simulink model "VCU_CS75_10_9_SteeringTorque"  (R2014a)
settings: Solver=FixedStepDiscrete  StartTime=0.0  StopTime=25  FixedStep=0.0005  RelTol=1e-3
undefined symbols (not defined in the file or in its folder): AutoDrivingReady, ecucoder_acal, I_SW01_L, LaterlAngleCommand, LDW, RemoteAcclPosition
libraries: simulink x880, ec5744lib x37
(part 15 of 30)

== system VCU_CS75_10_9_SteeringTorque/长安CS75底盘程序，20ms一次/Output/CAN1_Tx/to28D/LAS_28D/LAS_LDWReminder ==
  LAS_LDWReminder : Inport
  Constant{1..2,4..8} (7 alike) : Constant  Value=0  OutDataTypeStr=uint8
  LAS_LDWReminderRon : Rounding  Operator=round
  LAS_LDWReminder_1sat : Saturate  UpperLimit=96  LowerLimit=0
  LAS_LDWReminder_Convert : DataTypeConversion  OutDataTypeStr=uint8
  LAS_LDWReminder_Convert1 : DataTypeConversion  OutDataTypeStr=uint32
  LAS_LDWReminder_D : Product  Inputs=*/
  LAS_LDWReminder_F : Constant  OutDataTypeStr=single
  LAS_LDWReminder_L : simulink/Logic and Bit Operations/Bitwise Operator  logicop=AND  UseBitMask=on  BitMask=96  BitMaskRealWorld=Stored Integer
  LAS_LDWReminder_O : Constant  Value=0  OutDataTypeStr=single
  LAS_LDWReminder_S : ArithShift  BitShiftNumber=-5
  LAS_LDWReminder_sat : Saturate  UpperLimit=0  LowerLimit=0
  LAS_LDWReminder_st : Sum  Inputs=+-
  output1 : Outport
  output2 : Outport  Port=2
  output3 : Outport  Port=3
  output4 : Outport  Port=4
  output5 : Outport  Port=5
  output6 : Outport  Port=6
  output7 : Outport  Port=7
  output8 : Outport  Port=8
  wires:
  LAS_LDWReminder/1 -> LAS_LDWReminder_sat/1
  LAS_LDWReminder_sat/1 -> LAS_LDWReminder_st/1
  LAS_LDWReminder_O/1 -> LAS_LDWReminder_st/2
  LAS_LDWReminder_st/1 -> LAS_LDWReminder_D/1
  LAS_LDWReminder_F/1 -> LAS_LDWReminder_D/2
  LAS_LDWReminder_D/1 -> LAS_LDWReminderRon/1
  LAS_LDWReminderRon/1 -> LAS_LDWReminder_S/1
  LAS_LDWReminder_S/1 -> LAS_LDWReminder_1sat/1
  LAS_LDWReminder_1sat/1 -> LAS_LDWReminder_Convert1/1
  LAS_LDWReminder_Convert1/1 -> LAS_LDWReminder_L/1
  LAS_LDWReminder_L/1 -> LAS_LDWReminder_Convert/1
  LAS_LDWReminder_Convert/1 -> output3/1
  Constant1/1 -> output1/1
  Constant2/1 -> output2/1
  Constant4/1 -> output4/1
  Constant5/1 -> output5/1
  Constant6/1 -> output6/1
  Constant7/1 -> output7/1
  Constant8/1 -> output8/1

== system VCU_CS75_10_9_SteeringTorque/长安CS75底盘程序，20ms一次/Output/CAN1_Tx/to28D/LAS_28D/LAS_LDWStatus ==
  LAS_LDWStatus : Inport
  Constant{2..8} (7 alike) : Constant  Value=0  OutDataTypeStr=uint8
  LAS_LDWStatusRon : Rounding  Operator=round
  LAS_LDWStatus_1sat : Saturate  UpperLimit=96  LowerLimit=0
  LAS_LDWStatus_Convert : DataTypeConversion  OutDataTypeStr=uint8
  LAS_LDWStatus_Convert1 : DataTypeConversion  OutDataTypeStr=uint32
  LAS_LDWStatus_D : Product  Inputs=*/
  LAS_LDWStatus_F : Constant  OutDataTypeStr=single
  LAS_LDWStatus_L : simulink/Logic and Bit Operations/Bitwise Operator  logicop=AND  UseBitMask=on  BitMask=96  BitMaskRealWorld=Stored Integer
  LAS_LDWStatus_O : Constant  Value=0  OutDataTypeStr=single
  LAS_LDWStatus_S : ArithShift  BitShiftNumber=-5
  LAS_LDWStatus_sat : Saturate  UpperLimit=3  LowerLimit=0
  LAS_LDWStatus_st : Sum  Inputs=+-
  output1 : Outport
  output2 : Outport  Port=2
  output3 : Outport  Port=3
  output4 : Outport  Port=4
  output5 : Outport  Port=5
  output6 : Outport  Port=6
  output7 : Outport  Port=7
  output8 : Outport  Port=8
  wires:
  LAS_LDWStatus/1 -> LAS_LDWStatus_sat/1
  LAS_LDWStatus_sat/1 -> LAS_LDWStatus_st/1
  LAS_LDWStatus_O/1 -> LAS_LDWStatus_st/2
  LAS_LDWStatus_st/1 -> LAS_LDWStatus_D/1
  LAS_LDWStatus_F/1 -> LAS_LDWStatus_D/2
  LAS_LDWStatus_D/1 -> LAS_LDWStatusRon/1
  LAS_LDWStatusRon/1 -> LAS_LDWStatus_S/1
  LAS_LDWStatus_S/1 -> LAS_LDWStatus_1sat/1
  LAS_LDWStatus_1sat/1 -> LAS_LDWStatus_Convert1/1
  LAS_LDWStatus_Convert1/1 -> LAS_LDWStatus_L/1
  LAS_LDWStatus_L/1 -> LAS_LDWStatus_Convert/1
  LAS_LDWStatus_Convert/1 -> output1/1
  Constant2/1 -> output2/1
  Constant3/1 -> output3/1
  Constant4/1 -> output4/1
  Constant5/1 -> output5/1
  Constant6/1 -> output6/1
  Constant7/1 -> output7/1
  Constant8/1 -> output8/1

== system VCU_CS75_10_9_SteeringTorque/长安CS75底盘程序，20ms一次/Output/CAN1_Tx/to28D/LAS_28D/LAS_LDWVibrationWarning ==
  LAS_LDWVibrationWarning : Inport
  Constant{1,3..8} (7 alike) : Constant  Value=0  OutDataTypeStr=uint8
  LAS_LDWVibrationWarningRon : Rounding  Operator=round
  LAS_LDWVibrationWarning_1sat : Saturate  UpperLimit=96  LowerLimit=0
  LAS_LDWVibrationWarning_Convert : DataTypeConversion  OutDataTypeStr=uint8
  LAS_LDWVibrationWarning_Convert1 : DataTypeConversion  OutDataTypeStr=uint32
  LAS_LDWVibrationWarning_D : Product  Inputs=*/
  LAS_LDWVibrationWarning_F : Constant  OutDataTypeStr=single
  LAS_LDWVibrationWarning_L : simulink/Logic and Bit Operations/Bitwise Operator  logicop=AND  UseBitMask=on  BitMask=96  BitMaskRealWorld=Stored Integer
  LAS_LDWVibrationWarning_O : Constant  Value=0  OutDataTypeStr=single
  LAS_LDWVibrationWarning_S : ArithShift  BitShiftNumber=-5
  LAS_LDWVibrationWarning_sat : Saturate  UpperLimit=3  LowerLimit=0
  LAS_LDWVibrationWarning_st : Sum  Inputs=+-
  output1 : Outport
  output2 : Outport  Port=2
  output3 : Outport  Port=3
  output4 : Outport  Port=4
  output5 : Outport  Port=5
  output6 : Outport  Port=6
  output7 : Outport  Port=7
  output8 : Outport  Port=8
  wires:
  LAS_LDWVibrationWarning/1 -> LAS_LDWVibrationWarning_sat/1
  LAS_LDWVibrationWarning_sat/1 -> LAS_LDWVibrationWarning_st/1
  LAS_LDWVibrationWarning_O/1 -> LAS_LDWVibrationWarning_st/2
  LAS_LDWVibrationWarning_st/1 -> LAS_LDWVibrationWarning_D/1
  LAS_LDWVibrationWarning_F/1 -> LAS_LDWVibrationWarning_D/2
  LAS_LDWVibrationWarning_D/1 -> LAS_LDWVibrationWarningRon/1
  LAS_LDWVibrationWarningRon/1 -> LAS_LDWVibrationWarning_S/1
  LAS_LDWVibrationWarning_S/1 -> LAS_LDWVibrationWarning_1sat/1
  LAS_LDWVibrationWarning_1sat/1 -> LAS_LDWVibrationWarning_Convert1/1
  LAS_LDWVibrationWarning_Convert1/1 -> LAS_LDWVibrationWarning_L/1
  LAS_LDWVibrationWarning_L/1 -> LAS_LDWVibrationWarning_Convert/1
  LAS_LDWVibrationWarning_Convert/1 -> output2/1
  Constant1/1 -> output1/1
  Constant3/1 -> output3/1
  Constant4/1 -> output4/1
  Constant5/1 -> output5/1
  Constant6/1 -> output6/1
  Constant7/1 -> output7/1
  Constant8/1 -> output8/1

== system VCU_CS75_10_9_SteeringTorque/长安CS75底盘程序，20ms一次/Output/CAN1_Tx/to28D/LAS_28D/LAS_LKSStatus ==
  LAS_LKSStatus : Inport
  Constant{1..4,6..8} (7 alike) : Constant  Value=0  OutDataTypeStr=uint8
  LAS_LKSStatusRon : Rounding  Operator=round
  LAS_LKSStatus_1sat : Saturate  UpperLimit=224  LowerLimit=0
  LAS_LKSStatus_Convert : DataTypeConversion  OutDataTypeStr=uint8
  LAS_LKSStatus_Convert1 : DataTypeConversion  OutDataTypeStr=uint32
  LAS_LKSStatus_D : Product  Inputs=*/
  LAS_LKSStatus_F : Constant  OutDataTypeStr=single
  LAS_LKSStatus_L : simulink/Logic and Bit Operations/Bitwise Operator  logicop=AND  UseBitMask=on  BitMask=224  BitMaskRealWorld=Stored Integer
  LAS_LKSStatus_O : Constant  Value=0  OutDataTypeStr=single
  LAS_LKSStatus_S : ArithShift  BitShiftNumber=-5
  LAS_LKSStatus_sat : Saturate  UpperLimit=7  LowerLimit=0
  LAS_LKSStatus_st : Sum  Inputs=+-
  output1 : Outport
  output2 : Outport  Port=2
  output3 : Outport  Port=3
  output4 : Outport  Port=4
  output5 : Outport  Port=5
  output6 : Outport  Port=6
  output7 : Outport  Port=7
  output8 : Outport  Port=8
  wires:
  LAS_LKSStatus/1 -> LAS_LKSStatus_sat/1
  LAS_LKSStatus_sat/1 -> LAS_LKSStatus_st/1
  LAS_LKSStatus_O/1 -> LAS_LKSStatus_st/2
  LAS_LKSStatus_st/1 -> LAS_LKSStatus_D/1
  LAS_LKSStatus_F/1 -> LAS_LKSStatus_D/2
  LAS_LKSStatus_D/1 -> LAS_LKSStatusRon/1
  LAS_LKSStatusRon/1 -> LAS_LKSStatus_S/1
  LAS_LKSStatus_S/1 -> LAS_LKSStatus_1sat/1
  LAS_LKSStatus_1sat/1 -> LAS_LKSStatus_Convert1/1
  LAS_LKSStatus_Convert1/1 -> LAS_LKSStatus_L/1
  LAS_LKSStatus_L/1 -> LAS_LKSStatus_Convert/1
  LAS_LKSStatus_Convert/1 -> output5/1
  Constant1/1 -> output1/1
  Constant2/1 -> output2/1
  Constant3/1 -> output3/1
  Constant4/1 -> output4/1
  Constant6/1 -> output6/1
  Constant7/1 -> output7/1
  Constant8/1 -> output8/1

== system VCU_CS75_10_9_SteeringTorque/长安CS75底盘程序，20ms一次/Output/CAN1_Tx/to28D/LAS_28D/LAS_SLASpdLimit ==
  LAS_SLASpdLimit : Inport
  Constant{1..2,5..8} (6 alike) : Constant  Value=0  OutDataTypeStr=uint8
  LAS_SLASpdLimitBitCov : DataTypeConversion  OutDataTypeStr=uint8
  LAS_SLASpdLimitCOV : DataTypeConversion  OutDataTypeStr=uint8
  LAS_SLASpdLimitRon : Rounding  Operator=round
  LAS_SLASpdLimit_1sat : Saturate  UpperLimit=4080  LowerLimit=0
  LAS_SLASpdLimit_And : simulink/Logic and Bit Operations/Bitwise Operator  logicop=AND  UseBitMask=off  NumInputPorts=2  BitMask=bin2dec('11011001')  BitMaskRealWorld=Stored Integer
  LAS_SLASpdLimit_And_C : Constant  Value=255  OutDataTypeStr=uint32
  LAS_SLASpdLimit_Convert : DataTypeConversion  OutDataTypeStr=uint32
  LAS_SLASpdLimit_D : Product  Inputs=*/
  LAS_SLASpdLimit_D1 : Product  Inputs=*/
  LAS_SLASpdLimit_F : Constant  OutDataTypeStr=single
  LAS_SLASpdLimit_L : simulink/Logic and Bit Operations/Bitwise Operator  logicop=AND  UseBitMask=on  BitMask=4080  BitMaskRealWorld=Stored Integer
  LAS_SLASpdLimit_O : Constant  Value=0  OutDataTypeStr=single
  LAS_SLASpdLimit_S : ArithShift  BitShiftNumber=-4
  LAS_SLASpdLimit_sat : Saturate  UpperLimit=0  LowerLimit=0
  LAS_SLASpdLimit_st : Sum  Inputs=+-
  LAS_SLASpdLimitoutput3_C : Constant  Value=256
  output1 : Outport
  output2 : Outport  Port=2
  output3 : Outport  Port=3
  output4 : Outport  Port=4
  output5 : Outport  Port=5
  output6 : Outport  Port=6
  output7 : Outport  Port=7
  output8 : Outport  Port=8
  wires:
  LAS_SLASpdLimit/1 -> LAS_SLASpdLimit_sat/1
  LAS_SLASpdLimit_sat/1 -> LAS_SLASpdLimit_st/1
  LAS_SLASpdLimit_O/1 -> LAS_SLASpdLimit_st/2
  LAS_SLASpdLimit_st/1 -> LAS_SLASpdLimit_D/1
  LAS_SLASpdLimit_F/1 -> LAS_SLASpdLimit_D/2
  LAS_SLASpdLimit_D/1 -> LAS_SLASpdLimitRon/1
  LAS_SLASpdLimitRon/1 -> LAS_SLASpdLimit_S/1
  LAS_SLASpdLimit_S/1 -> LAS_SLASpdLimit_1sat/1
  LAS_SLASpdLimit_1sat/1 -> LAS_SLASpdLimit_Convert/1
  LAS_SLASpdLimit_Convert/1 -> LAS_SLASpdLimit_L/1
  LAS_SLASpdLimit_L/1 -> LAS_SLASpdLimit_D1/1, LAS_SLASpdLimit_And/1
  LAS_SLASpdLimitoutput3_C/1 -> LAS_SLASpdLimit_D1/2
  LAS_SLASpdLimit_D1/1 -> LAS_SLASpdLimitCOV/1
  LAS_SLASpdLimitCOV/1 -> output3/1
  LAS_SLASpdLimit_And_C/1 -> LAS_SLASpdLimit_And/2
  LAS_SLASpdLimit_And/1 -> LAS_SLASpdLimitBitCov/1
  LAS_SLASpdLimitBitCov/1 -> output4/1
  Constant1/1 -> output1/1
  Constant2/1 -> output2/1
  Constant5/1 -> output5/1
  Constant6/1 -> output6/1
  Constant7/1 -> output7/1
  Constant8/1 -> output8/1

== system VCU_CS75_10_9_SteeringTorque/长安CS75底盘程序，20ms一次/Output/CAN1_Tx/to28D/LAS_28D/LAS_SLASpdLimitUnit ==
  LAS_SLASpdLimitUnit : Inport
  Constant{2..8} (7 alike) : Constant  Value=0  OutDataTypeStr=uint8
  LAS_SLASpdLimitUnitRon : Rounding  Operator=round
  LAS_SLASpdLimitUnit_1sat : Saturate  UpperLimit=12  LowerLimit=0
  LAS_SLASpdLimitUnit_Convert : DataTypeConversion  OutDataTypeStr=uint8
  LAS_SLASpdLimitUnit_Convert1 : DataTypeConversion  OutDataTypeStr=uint32
  LAS_SLASpdLimitUnit_D : Product  Inputs=*/
  LAS_SLASpdLimitUnit_F : Constant  OutDataTypeStr=single
  LAS_SLASpdLimitUnit_L : simulink/Logic and Bit Operations/Bitwise Operator  logicop=AND  UseBitMask=on  BitMask=12  BitMaskRealWorld=Stored Integer
  LAS_SLASpdLimitUnit_O : Constant  Value=0  OutDataTypeStr=single
  LAS_SLASpdLimitUnit_S : ArithShift  BitShiftNumber=-2
  LAS_SLASpdLimitUnit_sat : Saturate  UpperLimit=0  LowerLimit=0
  LAS_SLASpdLimitUnit_st : Sum  Inputs=+-
  output1 : Outport
  output2 : Outport  Port=2
  output3 : Outport  Port=3
  output4 : Outport  Port=4
  output5 : Outport  Port=5
  output6 : Outport  Port=6
  output7 : Outport  Port=7
  output8 : Outport  Port=8
  wires:
  LAS_SLASpdLimitUnit/1 -> LAS_SLASpdLimitUnit_sat/1
  LAS_SLASpdLimitUnit_sat/1 -> LAS_SLASpdLimitUnit_st/1
  LAS_SLASpdLimitUnit_O/1 -> LAS_SLASpdLimitUnit_st/2
  LAS_SLASpdLimitUnit_st/1 -> LAS_SLASpdLimitUnit_D/1
  LAS_SLASpdLimitUnit_F/1 -> LAS_SLASpdLimitUnit_D/2
  LAS_SLASpdLimitUnit_D/1 -> LAS_SLASpdLimitUnitRon/1
  LAS_SLASpdLimitUnitRon/1 -> LAS_SLASpdLimitUnit_S/1
  LAS_SLASpdLimitUnit_S/1 -> LAS_SLASpdLimitUnit_1sat/1
  LAS_SLASpdLimitUnit_1sat/1 -> LAS_SLASpdLimitUnit_Convert1/1
  LAS_SLASpdLimitUnit_Convert1/1 -> LAS_SLASpdLimitUnit_L/1
  LAS_SLASpdLimitUnit_L/1 -> LAS_SLASpdLimitUnit_Convert/1
  LAS_SLASpdLimitUnit_Convert/1 -> output1/1
  Constant2/1 -> output2/1
  Constant3/1 -> output3/1
  Constant4/1 -> output4/1
  Constant5/1 -> output5/1
  Constant6/1 -> output6/1
  Constant7/1 -> output7/1
  Constant8/1 -> output8/1

== system VCU_CS75_10_9_SteeringTorque/长安CS75底盘程序，20ms一次/Output/CAN1_Tx/to28D/LAS_28D/LAS_SLAState ==
  LAS_SLAState : Inport
  Constant{1..4,6..8} (7 alike) : Constant  Value=0  OutDataTypeStr=uint8
  LAS_SLAStateRon : Rounding  Operator=round
  LAS_SLAState_1sat : Saturate  UpperLimit=28  LowerLimit=0
  LAS_SLAState_Convert : DataTypeConversion  OutDataTypeStr=uint8
  LAS_SLAState_Convert1 : DataTypeConversion  OutDataTypeStr=uint32
  LAS_SLAState_D : Product  Inputs=*/
  LAS_SLAState_F : Constant  OutDataTypeStr=single
  LAS_SLAState_L : simulink/Logic and Bit Operations/Bitwise Operator  logicop=AND  UseBitMask=on  BitMask=28  BitMaskRealWorld=Stored Integer
  LAS_SLAState_O : Constant  Value=0  OutDataTypeStr=single
  LAS_SLAState_S : ArithShift  BitShiftNumber=-2
  LAS_SLAState_sat : Saturate  UpperLimit=0  LowerLimit=0
  LAS_SLAState_st : Sum  Inputs=+-
  output1 : Outport
  output2 : Outport  Port=2
  output3 : Outport  Port=3
  output4 : Outport  Port=4
  output5 : Outport  Port=5
  output6 : Outport  Port=6
  output7 : Outport  Port=7
  output8 : Outport  Port=8
  wires:
  LAS_SLAState/1 -> LAS_SLAState_sat/1
  LAS_SLAState_sat/1 -> LAS_SLAState_st/1
  LAS_SLAState_O/1 -> LAS_SLAState_st/2
  LAS_SLAState_st/1 -> LAS_SLAState_D/1
  LAS_SLAState_F/1 -> LAS_SLAState_D/2
  LAS_SLAState_D/1 -> LAS_SLAStateRon/1
  LAS_SLAStateRon/1 -> LAS_SLAState_S/1
  LAS_SLAState_S/1 -> LAS_SLAState_1sat/1
  LAS_SLAState_1sat/1 -> LAS_SLAState_Convert1/1
  LAS_SLAState_Convert1/1 -> LAS_SLAState_L/1
  LAS_SLAState_L/1 -> LAS_SLAState_Convert/1
  LAS_SLAState_Convert/1 -> output5/1
  Constant1/1 -> output1/1
  Constant2/1 -> output2/1
  Constant3/1 -> output3/1
  Constant4/1 -> output4/1
  Constant6/1 -> output6/1
  Constant7/1 -> output7/1
  Constant8/1 -> output8/1

== system VCU_CS75_10_9_SteeringTorque/长安CS75底盘程序，20ms一次/Output/CAN1_Tx/to28D/LAS_28D/LAS_SteeringTorqueReq ==
  LAS_SteeringTorqueReq : Inport
  Constant{1..4,8} (5 alike) : Constant  Value=0  OutDataTypeStr=uint8
  LAS_SteeringTorqueReqBitCov : DataTypeConversion  OutDataTypeStr=uint32
  LAS_SteeringTorqueReqBitCov1 : DataTypeConversion  OutDataTypeStr=uint8
  LAS_SteeringTorqueReqCOV : DataTypeConversion  OutDataTypeStr=uint8
  LAS_SteeringTorqueReqCOV1 : DataTypeConversion  OutDataTypeStr=uint8
  LAS_SteeringTorqueReqRon : Rounding  Operator=round
  LAS_SteeringTorqueReq_1sat : Saturate  UpperLimit=262016  LowerLimit=0
  LAS_SteeringTorqueReq_And : simulink/Logic and Bit Operations/Bitwise Operator  logicop=AND  UseBitMask=off  NumInputPorts=2  BitMask=bin2dec('11011001')  BitMaskRealWorld=Stored Integer
  LAS_SteeringTorqueReq_And1 : simulink/Logic and Bit Operations/Bitwise Operator  logicop=AND  UseBitMask=off  NumInputPorts=2  BitMask=bin2dec('11011001')  BitMaskRealWorld=Stored Integer
  LAS_SteeringTorqueReq_And1_C : Constant  Value=255  OutDataTypeStr=uint32
  LAS_SteeringTorqueReq_And_C : Constant  Value=65535
  LAS_SteeringTorqueReq_Convert : DataTypeConversion  OutDataTypeStr=uint32
  LAS_SteeringTorqueReq_D : Product  Inputs=*/
  LAS_SteeringTorqueReq_D1 : Product  Inputs=*/
  LAS_SteeringTorqueReq_D2 : Product  Inputs=*/
  LAS_SteeringTorqueReq_F : Constant  Value=0.01  OutDataTypeStr=single
  LAS_SteeringTorqueReq_L : simulink/Logic and Bit Operations/Bitwise Operator  logicop=AND  UseBitMask=on  BitMask=262016  BitMaskRealWorld=Stored Integer
  LAS_SteeringTorqueReq_O : Constant  Value=-8  OutDataTypeStr=single
  LAS_SteeringTorqueReq_S : ArithShift  BitShiftNumber=-7
  LAS_SteeringTorqueReq_sat : Saturate  UpperLimit=12.47  LowerLimit=-8
  LAS_SteeringTorqueReq_st : Sum  Inputs=+-
  LAS_SteeringTorqueReqoutput5_C : Constant  Value=65536
  LAS_SteeringTorqueReqoutput6_C : Constant  Value=256
  output1 : Outport
  output2 : Outport  Port=2
  output3 : Outport  Port=3
  output4 : Outport  Port=4
  output5 : Outport  Port=5
  output6 : Outport  Port=6
  output7 : Outport  Port=7
  output8 : Outport  Port=8
  wires:
  LAS_SteeringTorqueReq/1 -> LAS_SteeringTorqueReq_sat/1
  LAS_SteeringTorqueReq_sat/1 -> LAS_SteeringTorqueReq_st/1
  LAS_SteeringTorqueReq_O/1 -> LAS_SteeringTorqueReq_st/2
  LAS_SteeringTorqueReq_st/1 -> LAS_SteeringTorqueReq_D/1
  LAS_SteeringTorqueReq_F/1 -> LAS_SteeringTorqueReq_D/2
  LAS_SteeringTorqueReq_D/1 -> LAS_SteeringTorqueReqRon/1
  LAS_SteeringTorqueReqRon/1 -> LAS_SteeringTorqueReq_S/1
  LAS_SteeringTorqueReq_S/1 -> LAS_SteeringTorqueReq_1sat/1
  LAS_SteeringTorqueReq_1sat/1 -> LAS_SteeringTorqueReq_Convert/1
  LAS_SteeringTorqueReq_Convert/1 -> LAS_SteeringTorqueReq_L/1
  LAS_SteeringTorqueReq_L/1 -> LAS_SteeringTorqueReq_D1/1, LAS_SteeringTorqueReq_And/1, LAS_SteeringTorqueReq_And1/1
  LAS_SteeringTorqueReqoutput5_C/1 -> LAS_SteeringTorqueReq_D1/2
  LAS_SteeringTorqueReq_D1/1 -> LAS_SteeringTorqueReqCOV/1
  LAS_SteeringTorqueReqCOV/1 -> output5/1
  LAS_SteeringTorqueReq_And_C/1 -> LAS_SteeringTorqueReqBitCov/1
  LAS_SteeringTorqueReqBitCov/1 -> LAS_SteeringTorqueReq_And/2
  LAS_SteeringTorqueReq_And/1 -> LAS_SteeringTorqueReq_D2/1
  LAS_SteeringTorqueReqoutput6_C/1 -> LAS_SteeringTorqueReq_D2/2
  LAS_SteeringTorqueReq_D2/1 -> LAS_SteeringTorqueReqCOV1/1
  LAS_SteeringTorqueReqCOV1/1 -> output6/1
  LAS_SteeringTorqueReq_And1_C/1 -> LAS_SteeringTorqueReq_And1/2
  LAS_SteeringTorqueReq_And1/1 -> LAS_SteeringTorqueReqBitCov1/1
  LAS_SteeringTorqueReqBitCov1/1 -> output7/1
  Constant1/1 -> output1/1
  Constant2/1 -> output2/1
  Constant3/1 -> output3/1
  Constant4/1 -> output4/1
  Constant8/1 -> output8/1

== system VCU_CS75_10_9_SteeringTorque/长安CS75底盘程序，20ms一次/Output/CAN1_Tx/to28D/LAS_28D/LAS_TakeoverReq ==
  LAS_TakeoverReq : Inport
  Constant{1,3..8} (7 alike) : Constant  Value=0  OutDataTypeStr=uint8
  LAS_TakeoverReqRon : Rounding  Operator=round
  LAS_TakeoverReq_1sat : Saturate  UpperLimit=4  LowerLimit=0
  LAS_TakeoverReq_Convert : DataTypeConversion  OutDataTypeStr=uint8
  LAS_TakeoverReq_Convert1 : DataTypeConversion  OutDataTypeStr=uint32
  LAS_TakeoverReq_D : Product  Inputs=*/
  LAS_TakeoverReq_F : Constant  OutDataTypeStr=single
  LAS_TakeoverReq_L : simulink/Logic and Bit Operations/Bitwise Operator  logicop=AND  UseBitMask=on  BitMask=4  BitMaskRealWorld=Stored Integer
  LAS_TakeoverReq_O : Constant  Value=0  OutDataTypeStr=single
  LAS_TakeoverReq_S : ArithShift  BitShiftNumber=-2
  LAS_TakeoverReq_sat : Saturate  UpperLimit=1  LowerLimit=0
  LAS_TakeoverReq_st : Sum  Inputs=+-
  output1 : Outport
  output2 : Outport  Port=2
  output3 : Outport  Port=3
  output4 : Outport  Port=4
  output5 : Outport  Port=5
  output6 : Outport  Port=6
  output7 : Outport  Port=7
  output8 : Outport  Port=8
  wires:
  LAS_TakeoverReq/1 -> LAS_TakeoverReq_sat/1
  LAS_TakeoverReq_sat/1 -> LAS_TakeoverReq_st/1
  LAS_TakeoverReq_O/1 -> LAS_TakeoverReq_st/2
  LAS_TakeoverReq_st/1 -> LAS_TakeoverReq_D/1
  LAS_TakeoverReq_F/1 -> LAS_TakeoverReq_D/2
  LAS_TakeoverReq_D/1 -> LAS_TakeoverReqRon/1
  LAS_TakeoverReqRon/1 -> LAS_TakeoverReq_S/1
  LAS_TakeoverReq_S/1 -> LAS_TakeoverReq_1sat/1
  LAS_TakeoverReq_1sat/1 -> LAS_TakeoverReq_Convert1/1
  LAS_TakeoverReq_Convert1/1 -> LAS_TakeoverReq_L/1
  LAS_TakeoverReq_L/1 -> LAS_TakeoverReq_Convert/1
  LAS_TakeoverReq_Convert/1 -> output2/1
  Constant1/1 -> output1/1
  Constant3/1 -> output3/1
  Constant4/1 -> output4/1
  Constant5/1 -> output5/1
  Constant6/1 -> output6/1
  Constant7/1 -> output7/1
  Constant8/1 -> output8/1

== system VCU_CS75_10_9_SteeringTorque/长安CS75底盘程序，20ms一次/Output/CAN1_Tx/to28D/LAS_28D/RollingConter ==
  RollingConter : Inport
  Constant{1..6,8} (7 alike) : Constant  Value=0  OutDataTypeStr=uint8
  RollingConterRon : Rounding  Operator=round
  RollingConter_1sat : Saturate  UpperLimit=15  LowerLimit=0
  RollingConter_Convert : DataTypeConversion  OutDataTypeStr=uint8
  RollingConter_Convert1 : DataTypeConversion  OutDataTypeStr=uint32
  RollingConter_D : Product  Inputs=*/
  RollingConter_F : Constant  OutDataTypeStr=single
  RollingConter_L : simulink/Logic and Bit Operations/Bitwise Operator  logicop=AND  UseBitMask=on  BitMask=15  BitMaskRealWorld=Stored Integer
  RollingConter_O : Constant  Value=0  OutDataTypeStr=single
  RollingConter_S : ArithShift
  RollingConter_sat : Saturate  UpperLimit=15  LowerLimit=0
  RollingConter_st : Sum  Inputs=+-
  output1 : Outport
  output2 : Outport  Port=2
  output3 : Outport  Port=3
  output4 : Outport  Port=4
  output5 : Outport  Port=5
  output6 : Outport  Port=6
  output7 : Outport  Port=7
  output8 : Outport  Port=8
  wires:
  RollingConter/1 -> RollingConter_sat/1
  RollingConter_sat/1 -> RollingConter_st/1
  RollingConter_O/1 -> RollingConter_st/2
  RollingConter_st/1 -> RollingConter_D/1
  RollingConter_F/1 -> RollingConter_D/2
  RollingConter_D/1 -> RollingConterRon/1
  RollingConterRon/1 -> RollingConter_S/1
  RollingConter_S/1 -> RollingConter_1sat/1
  RollingConter_1sat/1 -> RollingConter_Convert1/1
  RollingConter_Convert1/1 -> RollingConter_L/1
  RollingConter_L/1 -> RollingConter_Convert/1
  RollingConter_Convert/1 -> output7/1
  Constant1/1 -> output1/1
  Constant2/1 -> output2/1
  Constant3/1 -> output3/1
  Constant4/1 -> output4/1
  Constant5/1 -> output5/1
  Constant6/1 -> output6/1
  Constant8/1 -> output8/1

== system VCU_CS75_10_9_SteeringTorque/长安CS75底盘程序，20ms一次/Output/CAN1_Tx/to2E4/ACC_2E4/ACC_ACCTargetAcceleration ==
  ACC_ACCTargetAcceleration : Inport
  ACC_ACCTargetAccelerationRon : Rounding  Operator=round
  ACC_ACCTargetAcceleration_1sat : Saturate  UpperLimit=255  LowerLimit=0
  ACC_ACCTargetAcceleration_Convert : DataTypeConversion  OutDataTypeStr=uint8
  ACC_ACCTargetAcceleration_Convert1 : DataTypeConversion  OutDataTypeStr=uint32
  ACC_ACCTargetAcceleration_D : Product  Inputs=*/
  ACC_ACCTargetAcceleration_F : Constant  Value=0.05  OutDataTypeStr=single
  ACC_ACCTargetAcceleration_L : simulink/Logic and Bit Operations/Bitwise Operator  logicop=AND  UseBitMask=on  BitMask=255  BitMaskRealWorld=Stored Integer
  ACC_ACCTargetAcceleration_O : Constant  Value=-5  OutDataTypeStr=single
  ACC_ACCTargetAcceleration_S : ArithShift
  ACC_ACCTargetAcceleration_sat : Saturate  UpperLimit=7.75  LowerLimit=-5
  ACC_ACCTargetAcceleration_st : Sum  Inputs=+-
  Constant{1,3..8} (7 alike) : Constant  Value=0  OutDataTypeStr=uint8
  output1 : Outport
  output2 : Outport  Port=2
  output3 : Outport  Port=3
  output4 : Outport  Port=4
  output5 : Outport  Port=5
  output6 : Outport  Port=6
  output7 : Outport  Port=7
  output8 : Outport  Port=8
  wires:
  ACC_ACCTargetAcceleration/1 -> ACC_ACCTargetAcceleration_sat/1
  ACC_ACCTargetAcceleration_sat/1 -> ACC_ACCTargetAcceleration_st/1
  ACC_ACCTargetAcceleration_O/1 -> ACC_ACCTargetAcceleration_st/2
  ACC_ACCTargetAcceleration_st/1 -> ACC_ACCTargetAcceleration_D/1
  ACC_ACCTargetAcceleration_F/1 -> ACC_ACCTargetAcceleration_D/2
  ACC_ACCTargetAcceleration_D/1 -> ACC_ACCTargetAccelerationRon/1
  ACC_ACCTargetAccelerationRon/1 -> ACC_ACCTargetAcceleration_S/1
  ACC_ACCTargetAcceleration_S/1 -> ACC_ACCTargetAcceleration_1sat/1
  ACC_ACCTargetAcceleration_1sat/1 -> ACC_ACCTargetAcceleration_Convert1/1
  ACC_ACCTargetAcceleration_Convert1/1 -> ACC_ACCTargetAcceleration_L/1
  ACC_ACCTargetAcceleration_L/1 -> ACC_ACCTargetAcceleration_Convert/1
  ACC_ACCTargetAcceleration_Convert/1 -> output2/1
  Constant1/1 -> output1/1
  Constant3/1 -> output3/1
  Constant4/1 -> output4/1
  Constant5/1 -> output5/1
  Constant6/1 -> output6/1
  Constant7/1 -> output7/1
  Constant8/1 -> output8/1

== system VCU_CS75_10_9_SteeringTorque/长安CS75底盘程序，20ms一次/Output/CAN1_Tx/to2E4/ACC_2E4/ACC_CDDAxEnable ==
  ACC_CDDAxEnable : Inport
  ACC_CDDAxEnableRon : Rounding  Operator=round
  ACC_CDDAxEnable_1sat : Saturate  UpperLimit=1  LowerLimit=0
  ACC_CDDAxEnable_Convert : DataTypeConversion  OutDataTypeStr=uint8
  ACC_CDDAxEnable_Convert1 : DataTypeConversion  OutDataTypeStr=uint32
  ACC_CDDAxEnable_D : Product  Inputs=*/
  ACC_CDDAxEnable_F : Constant  OutDataTypeStr=single
  ACC_CDDAxEnable_L : simulink/Logic and Bit Operations/Bitwise Operator  logicop=AND  UseBitMask=on  BitMask=1  BitMaskRealWorld=Stored Integer
  ACC_CDDAxEnable_O : Constant  Value=0  OutDataTypeStr=single
  ACC_CDDAxEnable_S : ArithShift
  ACC_CDDAxEnable_sat : Saturate  UpperLimit=1  LowerLimit=0
  ACC_CDDAxEnable_st : Sum  Inputs=+-
  Constant{2..8} (7 alike) : Constant  Value=0  OutDataTypeStr=uint8
  output1 : Outport
  output2 : Outport  Port=2
  output3 : Outport  Port=3
  output4 : Outport  Port=4
  output5 : Outport  Port=5
  output6 : Outport  Port=6
  output7 : Outport  Port=7
  output8 : Outport  Port=8
  wires:
  ACC_CDDAxEnable/1 -> ACC_CDDAxEnable_sat/1
  ACC_CDDAxEnable_sat/1 -> ACC_CDDAxEnable_st/1
  ACC_CDDAxEnable_O/1 -> ACC_CDDAxEnable_st/2
  ACC_CDDAxEnable_st/1 -> ACC_CDDAxEnable_D/1
  ACC_CDDAxEnable_F/1 -> ACC_CDDAxEnable_D/2
  ACC_CDDAxEnable_D/1 -> ACC_CDDAxEnableRon/1
  ACC_CDDAxEnableRon/1 -> ACC_CDDAxEnable_S/1
  ACC_CDDAxEnable_S/1 -> ACC_CDDAxEnable_1sat/1
  ACC_CDDAxEnable_1sat/1 -> ACC_CDDAxEnable_Convert1/1
  ACC_CDDAxEnable_Convert1/1 -> ACC_CDDAxEnable_L/1
  ACC_CDDAxEnable_L/1 -> ACC_CDDAxEnable_Convert/1
  ACC_CDDAxEnable_Convert/1 -> output1/1
  Constant2/1 -> output2/1
  Constant3/1 -> output3/1
  Constant4/1 -> output4/1
  Constant5/1 -> output5/1
  Constant6/1 -> output6/1
  Constant7/1 -> output7/1
  Constant8/1 -> output8/1

== system VCU_CS75_10_9_SteeringTorque/长安CS75底盘程序，20ms一次/Output/CAN1_Tx/to2E4/ACC_2E4/ACC_CheckSum_id ==
  ACC_CheckSum_id : Inport
  ACC_CheckSum_idRon : Rounding  Operator=round
  ACC_CheckSum_id_1sat : Saturate  UpperLimit=255  LowerLimit=0
  ACC_CheckSum_id_Convert : DataTypeConversion  OutDataTypeStr=uint8
  ACC_CheckSum_id_Convert1 : DataTypeConversion  OutDataTypeStr=uint32
  ACC_CheckSum_id_D : Product  Inputs=*/
  ACC_CheckSum_id_F : Constant  OutDataTypeStr=single
  ACC_CheckSum_id_L : simulink/Logic and Bit Operations/Bitwise Operator  logicop=AND  UseBitMask=on  BitMask=255  BitMaskRealWorld=Stored Integer
  ACC_CheckSum_id_O : Constant  Value=0  OutDataTypeStr=single
  ACC_CheckSum_id_S : ArithShift
  ACC_CheckSum_id_sat : Saturate  UpperLimit=255  LowerLimit=0
  ACC_CheckSum_id_st : Sum  Inputs=+-
  Constant{1..7} (7 alike) : Constant  Value=0  OutDataTypeStr=uint8
  output1 : Outport
  output2 : Outport  Port=2
  output3 : Outport  Port=3
  output4 : Outport  Port=4
  output5 : Outport  Port=5
  output6 : Outport  Port=6
  output7 : Outport  Port=7
  output8 : Outport  Port=8
  wires:
  ACC_CheckSum_id/1 -> ACC_CheckSum_id_sat/1
  ACC_CheckSum_id_sat/1 -> ACC_CheckSum_id_st/1
  ACC_CheckSum_id_O/1 -> ACC_CheckSum_id_st/2
  ACC_CheckSum_id_st/1 -> ACC_CheckSum_id_D/1
  ACC_CheckSum_id_F/1 -> ACC_CheckSum_id_D/2
  ACC_CheckSum_id_D/1 -> ACC_CheckSum_idRon/1
  ACC_CheckSum_idRon/1 -> ACC_CheckSum_id_S/1
  ACC_CheckSum_id_S/1 -> ACC_CheckSum_id_1sat/1
  ACC_CheckSum_id_1sat/1 -> ACC_CheckSum_id_Convert1/1
  ACC_CheckSum_id_Convert1/1 -> ACC_CheckSum_id_L/1
  ACC_CheckSum_id_L/1 -> ACC_CheckSum_id_Convert/1
  ACC_CheckSum_id_Convert/1 -> output8/1
  Constant1/1 -> output1/1
  Constant2/1 -> output2/1
  Constant3/1 -> output3/1
  Constant4/1 -> output4/1
  Constant5/1 -> output5/1
  Constant6/1 -> output6/1
  Constant7/1 -> output7/1

== system VCU_CS75_10_9_SteeringTorque/长安CS75底盘程序，20ms一次/Output/CAN1_Tx/to2E4/ACC_2E4/ACC_DecToStop ==
  ACC_DecToStop : Inport
  ACC_DecToStopRon : Rounding  Operator=round
  ACC_DecToStop_1sat : Saturate  UpperLimit=2  LowerLimit=0
  ACC_DecToStop_Convert : DataTypeConversion  OutDataTypeStr=uint8
  ACC_DecToStop_Convert1 : DataTypeConversion  OutDataTypeStr=uint32
  ACC_DecToStop_D : Product  Inputs=*/
  ACC_DecToStop_F : Constant  OutDataTypeStr=single
  ACC_DecToStop_L : simulink/Logic and Bit Operations/Bitwise Operator  logicop=AND  UseBitMask=on  BitMask=2  BitMaskRealWorld=Stored Integer
  ACC_DecToStop_O : Constant  Value=0  OutDataTypeStr=single
  ACC_DecToStop_S : ArithShift  BitShiftNumber=-1
  ACC_DecToStop_sat : Saturate  UpperLimit=1  LowerLimit=0
  ACC_DecToStop_st : Sum  Inputs=+-
  Constant{2..8} (7 alike) : Constant  Value=0  OutDataTypeStr=uint8
  output1 : Outport
  output2 : Outport  Port=2
  output3 : Outport  Port=3
  output4 : Outport  Port=4
  output5 : Outport  Port=5
  output6 : Outport  Port=6
  output7 : Outport  Port=7
  output8 : Outport  Port=8
  wires:
  ACC_DecToStop/1 -> ACC_DecToStop_sat/1
  ACC_DecToStop_sat/1 -> ACC_DecToStop_st/1
  ACC_DecToStop_O/1 -> ACC_DecToStop_st/2
  ACC_DecToStop_st/1 -> ACC_DecToStop_D/1
  ACC_DecToStop_F/1 -> ACC_DecToStop_D/2
  ACC_DecToStop_D/1 -> ACC_DecToStopRon/1
  ACC_DecToStopRon/1 -> ACC_DecToStop_S/1
  ACC_DecToStop_S/1 -> ACC_DecToStop_1sat/1
  ACC_DecToStop_1sat/1 -> ACC_DecToStop_Convert1/1
  ACC_DecToStop_Convert1/1 -> ACC_DecToStop_L/1
  ACC_DecToStop_L/1 -> ACC_DecToStop_Convert/1
  ACC_DecToStop_Convert/1 -> output1/1
  Constant2/1 -> output2/1
  Constant3/1 -> output3/1
  Constant4/1 -> output4/1
  Constant5/1 -> output5/1
  Constant6/1 -> output6/1
  Constant7/1 -> output7/1
  Constant8/1 -> output8/1

== system VCU_CS75_10_9_SteeringTorque/长安CS75底盘程序，20ms一次/Output/CAN1_Tx/to2E4/ACC_2E4/ACC_Driveoff_Request ==
  ACC_Driveoff_Request : Inport
  ACC_Driveoff_RequestRon : Rounding  Operator=round
  ACC_Driveoff_Request_1sat : Saturate  UpperLimit=4  LowerLimit=0
  ACC_Driveoff_Request_Convert : DataTypeConversion  OutDataTypeStr=uint8
  ACC_Driveoff_Request_Convert1 : DataTypeConversion  OutDataTypeStr=uint32
  ACC_Driveoff_Request_D : Product  Inputs=*/
  ACC_Driveoff_Request_F : Constant  OutDataTypeStr=single
  ACC_Driveoff_Request_L : simulink/Logic and Bit Operations/Bitwise Operator  logicop=AND  UseBitMask=on  BitMask=4  BitMaskRealWorld=Stored Integer
  ACC_Driveoff_Request_O : Constant  Value=0  OutDataTypeStr=single
  ACC_Driveoff_Request_S : ArithShift  BitShiftNumber=-2
  ACC_Driveoff_Request_sat : Saturate  UpperLimit=1  LowerLimit=0
  ACC_Driveoff_Request_st : Sum  Inputs=+-
  Constant{2..8} (7 alike) : Constant  Value=0  OutDataTypeStr=uint8
  output1 : Outport
  output2 : Outport  Port=2
  output3 : Outport  Port=3
  output4 : Outport  Port=4
  output5 : Outport  Port=5
  output6 : Outport  Port=6
  output7 : Outport  Port=7
  output8 : Outport  Port=8
  wires:
  ACC_Driveoff_Request/1 -> ACC_Driveoff_Request_sat/1
  ACC_Driveoff_Request_sat/1 -> ACC_Driveoff_Request_st/1
  ACC_Driveoff_Request_O/1 -> ACC_Driveoff_Request_st/2
  ACC_Driveoff_Request_st/1 -> ACC_Driveoff_Request_D/1
  ACC_Driveoff_Request_F/1 -> ACC_Driveoff_Request_D/2
  ACC_Driveoff_Request_D/1 -> ACC_Driveoff_RequestRon/1
  ACC_Driveoff_RequestRon/1 -> ACC_Driveoff_Request_S/1
  ACC_Driveoff_Request_S/1 -> ACC_Driveoff_Request_1sat/1
  ACC_Driveoff_Request_1sat/1 -> ACC_Driveoff_Request_Convert1/1
  ACC_Driveoff_Request_Convert1/1 -> ACC_Driveoff_Request_L/1
  ACC_Driveoff_Request_L/1 -> ACC_Driveoff_Request_Convert/1
  ACC_Driveoff_Request_Convert/1 -> output1/1
  Constant2/1 -> output2/1
  Constant3/1 -> output3/1
  Constant4/1 -> output4/1
  Constant5/1 -> output5/1
  Constant6/1 -> output6/1
  Constant7/1 -> output7/1
  Constant8/1 -> output8/1

== system VCU_CS75_10_9_SteeringTorque/长安CS75底盘程序，20ms一次/Output/CAN1_Tx/to2E4/ACC_2E4/ACC_Mode ==
  ACC_Mode : Inport
  ACC_ModeRon : Rounding  Operator=round
  ACC_Mode_1sat : Saturate  UpperLimit=56  LowerLimit=0
  ACC_Mode_Convert : DataTypeConversion  OutDataTypeStr=uint8
  ACC_Mode_Convert1 : DataTypeConversion  OutDataTypeStr=uint32
  ACC_Mode_D : Product  Inputs=*/
  ACC_Mode_F : Constant  OutDataTypeStr=single
  ACC_Mode_L : simulink/Logic and Bit Operations/Bitwise Operator  logicop=AND  UseBitMask=on  BitMask=56  BitMaskRealWorld=Stored Integer
  ACC_Mode_O : Constant  Value=0  OutDataTypeStr=single
  ACC_Mode_S : ArithShift  BitShiftNumber=-3
  ACC_Mode_sat : Saturate  UpperLimit=7  LowerLimit=0
  ACC_Mode_st : Sum  Inputs=+-
  Constant{2..8} (7 alike) : Constant  Value=0  OutDataTypeStr=uint8
  output1 : Outport
  output2 : Outport  Port=2
  output3 : Outport  Port=3
  output4 : Outport  Port=4
  output5 : Outport  Port=5
  output6 : Outport  Port=6
  output7 : Outport  Port=7
  output8 : Outport  Port=8
  wires:
  ACC_Mode/1 -> ACC_Mode_sat/1
  ACC_Mode_sat/1 -> ACC_Mode_st/1
  ACC_Mode_O/1 -> ACC_Mode_st/2
  ACC_Mode_st/1 -> ACC_Mode_D/1
  ACC_Mode_F/1 -> ACC_Mode_D/2
  ACC_Mode_D/1 -> ACC_ModeRon/1
  ACC_ModeRon/1 -> ACC_Mode_S/1
  ACC_Mode_S/1 -> ACC_Mode_1sat/1
  ACC_Mode_1sat/1 -> ACC_Mode_Convert1/1
  ACC_Mode_Convert1/1 -> ACC_Mode_L/1
  ACC_Mode_L/1 -> ACC_Mode_Convert/1
  ACC_Mode_Convert/1 -> output1/1
  Constant2/1 -> output2/1
  Constant3/1 -> output3/1
  Constant4/1 -> output4/1
  Constant5/1 -> output5/1
  Constant6/1 -> output6/1
  Constant7/1 -> output7/1
  Constant8/1 -> output8/1

== system VCU_CS75_10_9_SteeringTorque/长安CS75底盘程序，20ms一次/Output/CAN1_Tx/to2E4/ACC_2E4/ACC_RollingCounter_id ==
  ACC_RollingCounter_id : Inport
  ACC_RollingCounter_idRon : Rounding  Operator=round
  ACC_RollingCounter_id_1sat : Saturate  UpperLimit=15  LowerLimit=0
  ACC_RollingCounter_id_Convert : DataTypeConversion  OutDataTypeStr=uint8
  ACC_RollingCounter_id_Convert1 : DataTypeConversion  OutDataTypeStr=uint32
  ACC_RollingCounter_id_D : Product  Inputs=*/
  ACC_RollingCounter_id_F : Constant  OutDataTypeStr=single
  ACC_RollingCounter_id_L : simulink/Logic and Bit Operations/Bitwise Operator  logicop=AND  UseBitMask=on  BitMask=15  BitMaskRealWorld=Stored Integer
  ACC_RollingCounter_id_O : Constant  Value=0  OutDataTypeStr=single
  ACC_RollingCounter_id_S : ArithShift
  ACC_RollingCounter_id_sat : Saturate  UpperLimit=15  LowerLimit=0
  ACC_RollingCounter_id_st : Sum  Inputs=+-
  Constant{1..6,8} (7 alike) : Constant  Value=0  OutDataTypeStr=uint8
  output1 : Outport
  output2 : Outport  Port=2
  output3 : Outport  Port=3
  output4 : Outport  Port=4
  output5 : Outport  Port=5
  output6 : Outport  Port=6
  output7 : Outport  Port=7
  output8 : Outport  Port=8
  wires:
  ACC_RollingCounter_id/1 -> ACC_RollingCounter_id_sat/1
  ACC_RollingCounter_id_sat/1 -> ACC_RollingCounter_id_st/1
  ACC_RollingCounter_id_O/1 -> ACC_RollingCounter_id_st/2
  ACC_RollingCounter_id_st/1 -> ACC_RollingCounter_id_D/1
  ACC_RollingCounter_id_F/1 -> ACC_RollingCounter_id_D/2
  ACC_RollingCounter_id_D/1 -> ACC_RollingCounter_idRon/1
  ACC_RollingCounter_idRon/1 -> ACC_RollingCounter_id_S/1
  ACC_RollingCounter_id_S/1 -> ACC_RollingCounter_id_1sat/1
  ACC_RollingCounter_id_1sat/1 -> ACC_RollingCounter_id_Convert1/1
  ACC_RollingCounter_id_Convert1/1 -> ACC_RollingCounter_id_L/1
  ACC_RollingCounter_id_L/1 -> ACC_RollingCounter_id_Convert/1
  ACC_RollingCounter_id_Convert/1 -> output7/1
  Constant1/1 -> output1/1
  Constant2/1 -> output2/1
  Constant3/1 -> output3/1
  Constant4/1 -> output4/1
  Constant5/1 -> output5/1
  Constant6/1 -> output6/1
  Constant8/1 -> output8/1

== system VCU_CS75_10_9_SteeringTorque/长安CS75底盘程序，20ms一次/Output/CAN1_Tx/to2E5/ACC_2E5/ACC_ABAavailable ==
  ACC_ABAavailable : Inport
  ACC_ABAavailableRon : Rounding  Operator=round
  ACC_ABAavailable_1sat : Saturate  UpperLimit=16  LowerLimit=0
  ACC_ABAavailable_Convert : DataTypeConversion  OutDataTypeStr=uint8
  ACC_ABAavailable_Convert1 : DataTypeConversion  OutDataTypeStr=uint32
  ACC_ABAavailable_D : Product  Inputs=*/
  ACC_ABAavailable_F : Constant  OutDataTypeStr=single
  ACC_ABAavailable_L : simulink/Logic and Bit Operations/Bitwise Operator  logicop=AND  UseBitMask=on  BitMask=16  BitMaskRealWorld=Stored Integer
  ACC_ABAavailable_O : Constant  Value=0  OutDataTypeStr=single
  ACC_ABAavailable_S : ArithShift  BitShiftNumber=-4
  ACC_ABAavailable_sat : Saturate  UpperLimit=1  LowerLimit=0
  ACC_ABAavailable_st : Sum  Inputs=+-
  Constant{1..2,4..8} (7 alike) : Constant  Value=0  OutDataTypeStr=uint8
  output1 : Outport
  output2 : Outport  Port=2
  output3 : Outport  Port=3
  output4 : Outport  Port=4
  output5 : Outport  Port=5
  output6 : Outport  Port=6
  output7 : Outport  Port=7
  output8 : Outport  Port=8
  wires:
  ACC_ABAavailable/1 -> ACC_ABAavailable_sat/1
  ACC_ABAavailable_sat/1 -> ACC_ABAavailable_st/1
  ACC_ABAavailable_O/1 -> ACC_ABAavailable_st/2
  ACC_ABAavailable_st/1 -> ACC_ABAavailable_D/1
  ACC_ABAavailable_F/1 -> ACC_ABAavailable_D/2
  ACC_ABAavailable_D/1 -> ACC_ABAavailableRon/1
  ACC_ABAavailableRon/1 -> ACC_ABAavailable_S/1
  ACC_ABAavailable_S/1 -> ACC_ABAavailable_1sat/1
  ACC_ABAavailable_1sat/1 -> ACC_ABAavailable_Convert1/1
  ACC_ABAavailable_Convert1/1 -> ACC_ABAavailable_L/1
  ACC_ABAavailable_L/1 -> ACC_ABAavailable_Convert/1
  ACC_ABAavailable_Convert/1 -> output3/1
  Constant1/1 -> output1/1
  Constant2/1 -> output2/1
  Constant4/1 -> output4/1
  Constant5/1 -> output5/1
  Constant6/1 -> output6/1
  Constant7/1 -> output7/1
  Constant8/1 -> output8/1

== system VCU_CS75_10_9_SteeringTorque/长安CS75底盘程序，20ms一次/Output/CAN1_Tx/to2E5/ACC_2E5/ACC_ABAlevel ==
  ACC_ABAlevel : Inport
  ACC_ABAlevelRon : Rounding  Operator=round
  ACC_ABAlevel_1sat : Saturate  UpperLimit=96  LowerLimit=0
  ACC_ABAlevel_Convert : DataTypeConversion  OutDataTypeStr=uint8
  ACC_ABAlevel_Convert1 : DataTypeConversion  OutDataTypeStr=uint32
  ACC_ABAlevel_D : Product  Inputs=*/
  ACC_ABAlevel_F : Constant  OutDataTypeStr=single
  ACC_ABAlevel_L : simulink/Logic and Bit Operations/Bitwise Operator  logicop=AND  UseBitMask=on  BitMask=96  BitMaskRealWorld=Stored Integer
  ACC_ABAlevel_O : Constant  Value=0  OutDataTypeStr=single
  ACC_ABAlevel_S : ArithShift  BitShiftNumber=-5
  ACC_ABAlevel_sat : Saturate  UpperLimit=3  LowerLimit=0
  ACC_ABAlevel_st : Sum  Inputs=+-
  Constant{1..4,6..8} (7 alike) : Constant  Value=0  OutDataTypeStr=uint8
  output1 : Outport
  output2 : Outport  Port=2
  output3 : Outport  Port=3
  output4 : Outport  Port=4
  output5 : Outport  Port=5
  output6 : Outport  Port=6
  output7 : Outport  Port=7
  output8 : Outport  Port=8
  wires:
  ACC_ABAlevel/1 -> ACC_ABAlevel_sat/1
  ACC_ABAlevel_sat/1 -> ACC_ABAlevel_st/1
  ACC_ABAlevel_O/1 -> ACC_ABAlevel_st/2
  ACC_ABAlevel_st/1 -> ACC_ABAlevel_D/1
  ACC_ABAlevel_F/1 -> ACC_ABAlevel_D/2
  ACC_ABAlevel_D/1 -> ACC_ABAlevelRon/1
  ACC_ABAlevelRon/1 -> ACC_ABAlevel_S/1
  ACC_ABAlevel_S/1 -> ACC_ABAlevel_1sat/1
  ACC_ABAlevel_1sat/1 -> ACC_ABAlevel_Convert1/1
  ACC_ABAlevel_Convert1/1 -> ACC_ABAlevel_L/1
  ACC_ABAlevel_L/1 -> ACC_ABAlevel_Convert/1
  ACC_ABAlevel_Convert/1 -> output5/1
  Constant1/1 -> output1/1
  Constant2/1 -> output2/1
  Constant3/1 -> output3/1
  Constant4/1 -> output4/1
  Constant6/1 -> output6/1
  Constant7/1 -> output7/1
  Constant8/1 -> output8/1

== system VCU_CS75_10_9_SteeringTorque/长安CS75底盘程序，20ms一次/Output/CAN1_Tx/to2E5/ACC_2E5/ACC_AEBDecCtrlAvail ==
  ACC_AEBDecCtrlAvail : Inport
  ACC_AEBDecCtrlAvailRon : Rounding  Operator=round
  ACC_AEBDecCtrlAvail_1sat : Saturate  UpperLimit=128  LowerLimit=0
  ACC_AEBDecCtrlAvail_Convert : DataTypeConversion  OutDataTypeStr=uint8
  ACC_AEBDecCtrlAvail_Convert1 : DataTypeConversion  OutDataTypeStr=uint32
  ACC_AEBDecCtrlAvail_D : Product  Inputs=*/
  ACC_AEBDecCtrlAvail_F : Constant  OutDataTypeStr=single
  ACC_AEBDecCtrlAvail_L : simulink/Logic and Bit Operations/Bitwise Operator  logicop=AND  UseBitMask=on  BitMask=128  BitMaskRealWorld=Stored Integer
  ACC_AEBDecCtrlAvail_O : Constant  Value=0  OutDataTypeStr=single
  ACC_AEBDecCtrlAvail_S : ArithShift  BitShiftNumber=-7
  ACC_AEBDecCtrlAvail_sat : Saturate  UpperLimit=1  LowerLimit=0
  ACC_AEBDecCtrlAvail_st : Sum  Inputs=+-
  Constant{1..4,6..8} (7 alike) : Constant  Value=0  OutDataTypeStr=uint8
  output1 : Outport
  output2 : Outport  Port=2
  output3 : Outport  Port=3
  output4 : Outport  Port=4
  output5 : Outport  Port=5
  output6 : Outport  Port=6
  output7 : Outport  Port=7
  output8 : Outport  Port=8
  wires:
  ACC_AEBDecCtrlAvail/1 -> ACC_AEBDecCtrlAvail_sat/1
  ACC_AEBDecCtrlAvail_sat/1 -> ACC_AEBDecCtrlAvail_st/1
  ACC_AEBDecCtrlAvail_O/1 -> ACC_AEBDecCtrlAvail_st/2
  ACC_AEBDecCtrlAvail_st/1 -> ACC_AEBDecCtrlAvail_D/1
  ACC_AEBDecCtrlAvail_F/1 -> ACC_AEBDecCtrlAvail_D/2
  ACC_AEBDecCtrlAvail_D/1 -> ACC_AEBDecCtrlAvailRon/1
  ACC_AEBDecCtrlAvailRon/1 -> ACC_AEBDecCtrlAvail_S/1
  ACC_AEBDecCtrlAvail_S/1 -> ACC_AEBDecCtrlAvail_1sat/1
  ACC_AEBDecCtrlAvail_1sat/1 -> ACC_AEBDecCtrlAvail_Convert1/1
  ACC_AEBDecCtrlAvail_Convert1/1 -> ACC_AEBDecCtrlAvail_L/1
  ACC_AEBDecCtrlAvail_L/1 -> ACC_AEBDecCtrlAvail_Convert/1
  ACC_AEBDecCtrlAvail_Convert/1 -> output5/1
  Constant1/1 -> output1/1
  Constant2/1 -> output2/1
  Constant3/1 -> output3/1
  Constant4/1 -> output4/1
  Constant6/1 -> output6/1
  Constant7/1 -> output7/1
  Constant8/1 -> output8/1

== system VCU_CS75_10_9_SteeringTorque/长安CS75底盘程序，20ms一次/Output/CAN1_Tx/to2E5/ACC_2E5/ACC_AEBLVehilcehold ==
  ACC_AEBLVehilcehold : Inport
  ACC_AEBLVehilceholdRon : Rounding  Operator=round
  ACC_AEBLVehilcehold_1sat : Saturate  UpperLimit=4  LowerLimit=0
  ACC_AEBLVehilcehold_Convert : DataTypeConversion  OutDataTypeStr=uint8
  ACC_AEBLVehilcehold_Convert1 : DataTypeConversion  OutDataTypeStr=uint32
  ACC_AEBLVehilcehold_D : Product  Inputs=*/
  ACC_AEBLVehilcehold_F : Constant  OutDataTypeStr=single
  ACC_AEBLVehilcehold_L : simulink/Logic and Bit Operations/Bitwise Operator  logicop=AND  UseBitMask=on  BitMask=4  BitMaskRealWorld=Stored Integer
  ACC_AEBLVehilcehold_O : Constant  Value=0  OutDataTypeStr=single
  ACC_AEBLVehilcehold_S : ArithShift  BitShiftNumber=-2
  ACC_AEBLVehilcehold_sat : Saturate  UpperLimit=1  LowerLimit=0
  ACC_AEBLVehilcehold_st : Sum  Inputs=+-
  Constant{1..3,5..8} (7 alike) : Constant  Value=0  OutDataTypeStr=uint8
  output1 : Outport
  output2 : Outport  Port=2
  output3 : Outport  Port=3
  output4 : Outport  Port=4
  output5 : Outport  Port=5
  output6 : Outport  Port=6
  output7 : Outport  Port=7
  output8 : Outport  Port=8
  wires:
  ACC_AEBLVehilcehold/1 -> ACC_AEBLVehilcehold_sat/1
  ACC_AEBLVehilcehold_sat/1 -> ACC_AEBLVehilcehold_st/1
  ACC_AEBLVehilcehold_O/1 -> ACC_AEBLVehilcehold_st/2
  ACC_AEBLVehilcehold_st/1 -> ACC_AEBLVehilcehold_D/1
  ACC_AEBLVehilcehold_F/1 -> ACC_AEBLVehilcehold_D/2
  ACC_AEBLVehilcehold_D/1 -> ACC_AEBLVehilceholdRon/1
  ACC_AEBLVehilceholdRon/1 -> ACC_AEBLVehilcehold_S/1
  ACC_AEBLVehilcehold_S/1 -> ACC_AEBLVehilcehold_1sat/1
  ACC_AEBLVehilcehold_1sat/1 -> ACC_AEBLVehilcehold_Convert1/1
  ACC_AEBLVehilcehold_Convert1/1 -> ACC_AEBLVehilcehold_L/1
  ACC_AEBLVehilcehold_L/1 -> ACC_AEBLVehilcehold_Convert/1
  ACC_AEBLVehilcehold_Convert/1 -> output4/1
  Constant1/1 -> output1/1
  Constant2/1 -> output2/1
  Constant3/1 -> output3/1
  Constant5/1 -> output5/1
  Constant6/1 -> output6/1
  Constant7/1 -> output7/1
  Constant8/1 -> output8/1

== system VCU_CS75_10_9_SteeringTorque/长安CS75底盘程序，20ms一次/Output/CAN1_Tx/to2E5/ACC_2E5/ACC_AEBTargetDeceleration ==
  ACC_AEBTargetDeceleration : Inport
  ACC_AEBTargetDecelerationBitCov : DataTypeConversion  OutDataTypeStr=uint32
  ACC_AEBTargetDecelerationBitCov1 : DataTypeConversion  OutDataTypeStr=uint8
  ACC_AEBTargetDecelerationCOV : DataTypeConversion  OutDataTypeStr=uint8
  ACC_AEBTargetDecelerationCOV1 : DataTypeConversion  OutDataTypeStr=uint8
  ACC_AEBTargetDecelerationRon : Rounding  Operator=round
  ACC_AEBTargetDeceleration_1sat : Saturate  UpperLimit=2097120  LowerLimit=0
  ACC_AEBTargetDeceleration_And : simulink/Logic and Bit Operations/Bitwise Operator  logicop=AND  UseBitMask=off  NumInputPorts=2  BitMask=bin2dec('11011001')  BitMaskRealWorld=Stored Integer
  ACC_AEBTargetDeceleration_And1 : simulink/Logic and Bit Operations/Bitwise Operator  logicop=AND  UseBitMask=off  NumInputPorts=2  BitMask=bin2dec('11011001')  BitMaskRealWorld=Stored Integer
  ACC_AEBTargetDeceleration_And1_C : Constant  Value=255  OutDataTypeStr=uint32
  ACC_AEBTargetDeceleration_And_C : Constant  Value=65535
  ACC_AEBTargetDeceleration_Convert : DataTypeConversion  OutDataTypeStr=uint32
  ACC_AEBTargetDeceleration_D : Product  Inputs=*/
  ACC_AEBTargetDeceleration_D1 : Product  Inputs=*/
  ACC_AEBTargetDeceleration_D2 : Product  Inputs=*/
  ACC_AEBTargetDeceleration_F : Constant  Value=0.0005  OutDataTypeStr=single
  ACC_AEBTargetDeceleration_L : simulink/Logic and Bit Operations/Bitwise Operator  logicop=AND  UseBitMask=on  BitMask=2097120  BitMaskRealWorld=Stored Integer
  ACC_AEBTargetDeceleration_O : Constant  Value=-16  OutDataTypeStr=single
  ACC_AEBTargetDeceleration_S : ArithShift  BitShiftNumber=-5
  ACC_AEBTargetDeceleration_sat : Saturate  UpperLimit=16  LowerLimit=-16
  ACC_AEBTargetDeceleration_st : Sum  Inputs=+-
  ACC_AEBTargetDecelerationoutput1_C : Constant  Value=65536
  ACC_AEBTargetDecelerationoutput2_C : Constant  Value=256
  Constant{4..8} (5 alike) : Constant  Value=0  OutDataTypeStr=uint8
  output1 : Outport
  output2 : Outport  Port=2
  output3 : Outport  Port=3
  output4 : Outport  Port=4
  output5 : Outport  Port=5
  output6 : Outport  Port=6
  output7 : Outport  Port=7
  output8 : Outport  Port=8
  wires:
  ACC_AEBTargetDeceleration/1 -> ACC_AEBTargetDeceleration_sat/1
  ACC_AEBTargetDeceleration_sat/1 -> ACC_AEBTargetDeceleration_st/1
  ACC_AEBTargetDeceleration_O/1 -> ACC_AEBTargetDeceleration_st/2
  ACC_AEBTargetDeceleration_st/1 -> ACC_AEBTargetDeceleration_D/1
  ACC_AEBTargetDeceleration_F/1 -> ACC_AEBTargetDeceleration_D/2
  ACC_AEBTargetDeceleration_D/1 -> ACC_AEBTargetDecelerationRon/1
  ACC_AEBTargetDecelerationRon/1 -> ACC_AEBTargetDeceleration_S/1
  ACC_AEBTargetDeceleration_S/1 -> ACC_AEBTargetDeceleration_1sat/1
  ACC_AEBTargetDeceleration_1sat/1 -> ACC_AEBTargetDeceleration_Convert/1
  ACC_AEBTargetDeceleration_Convert/1 -> ACC_AEBTargetDeceleration_L/1
  ACC_AEBTargetDeceleration_L/1 -> ACC_AEBTargetDeceleration_D1/1, ACC_AEBTargetDeceleration_And/1, ACC_AEBTargetDeceleration_And1/1
  ACC_AEBTargetDecelerationoutput1_C/1 -> ACC_AEBTargetDeceleration_D1/2
  ACC_AEBTargetDeceleration_D1/1 -> ACC_AEBTargetDecelerationCOV/1
  ACC_AEBTargetDecelerationCOV/1 -> output1/1
  ACC_AEBTargetDeceleration_And_C/1 -> ACC_AEBTargetDecelerationBitCov/1
  ACC_AEBTargetDecelerationBitCov/1 -> ACC_AEBTargetDeceleration_And/2
  ACC_AEBTargetDeceleration_And/1 -> ACC_AEBTargetDeceleration_D2/1
  ACC_AEBTargetDecelerationoutput2_C/1 -> ACC_AEBTargetDeceleration_D2/2
  ACC_AEBTargetDeceleration_D2/1 -> ACC_AEBTargetDecelerationCOV1/1
  ACC_AEBTargetDecelerationCOV1/1 -> output2/1
  ACC_AEBTargetDeceleration_And1_C/1 -> ACC_AEBTargetDeceleration_And1/2
  ACC_AEBTargetDeceleration_And1/1 -> ACC_AEBTargetDecelerationBitCov1/1
  ACC_AEBTargetDecelerationBitCov1/1 -> output3/1
  Constant4/1 -> output4/1
  Constant5/1 -> output5/1
  Constant6/1 -> output6/1
  Constant7/1 -> output7/1
  Constant8/1 -> output8/1

== system VCU_CS75_10_9_SteeringTorque/长安CS75底盘程序，20ms一次/Output/CAN1_Tx/to2E5/ACC_2E5/ACC_AWBavailable ==
  ACC_AWBavailable : Inport
  ACC_AWBavailableRon : Rounding  Operator=round
  ACC_AWBavailable_1sat : Saturate  UpperLimit=128  LowerLimit=0
  ACC_AWBavailable_Convert : DataTypeConversion  OutDataTypeStr=uint8
  ACC_AWBavailable_Convert1 : DataTypeConversion  OutDataTypeStr=uint32
  ACC_AWBavailable_D : Product  Inputs=*/
  ACC_AWBavailable_F : Constant  OutDataTypeStr=single
  ACC_AWBavailable_L : simulink/Logic and Bit Operations/Bitwise Operator  logicop=AND  UseBitMask=on  BitMask=128  BitMaskRealWorld=Stored Integer
  ACC_AWBavailable_O : Constant  Value=0  OutDataTypeStr=single
  ACC_AWBavailable_S : ArithShift  BitShiftNumber=-7
  ACC_AWBavailable_sat : Saturate  UpperLimit=1  LowerLimit=0
  ACC_AWBavailable_st : Sum  Inputs=+-
  Constant{1..3,5..8} (7 alike) : Constant  Value=0  OutDataTypeStr=uint8
  output1 : Outport
  output2 : Outport  Port=2
  output3 : Outport  Port=3
  output4 : Outport  Port=4
  output5 : Outport  Port=5
  output6 : Outport  Port=6
  output7 : Outport  Port=7
  output8 : Outport  Port=8
  wires:
  ACC_AWBavailable/1 -> ACC_AWBavailable_sat/1
  ACC_AWBavailable_sat/1 -> ACC_AWBavailable_st/1
  ACC_AWBavailable_O/1 -> ACC_AWBavailable_st/2
  ACC_AWBavailable_st/1 -> ACC_AWBavailable_D/1
  ACC_AWBavailable_F/1 -> ACC_AWBavailable_D/2
  ACC_AWBavailable_D/1 -> ACC_AWBavailableRon/1
  ACC_AWBavailableRon/1 -> ACC_AWBavailable_S/1
  ACC_AWBavailable_S/1 -> ACC_AWBavailable_1sat/1
  ACC_AWBavailable_1sat/1 -> ACC_AWBavailable_Convert1/1
  ACC_AWBavailable_Convert1/1 -> ACC_AWBavailable_L/1
  ACC_AWBavailable_L/1 -> ACC_AWBavailable_Convert/1
  ACC_AWBavailable_Convert/1 -> output4/1
  Constant1/1 -> output1/1
  Constant2/1 -> output2/1
  Constant3/1 -> output3/1
  Constant5/1 -> output5/1
  Constant6/1 -> output6/1
  Constant7/1 -> output7/1
  Constant8/1 -> output8/1
